simulink model "IEEE9_case"  (R2024b)
settings: Solver=FixedStepAuto  StartTime=0  StopTime=5  FixedStep=1e-7  RelTol=1e-3
values from neighbouring files (symbols this model uses):
  SG_D_1_D = 0.01056    [IEEE9_case_parameters.m]    (also in case1_parameters.m; case2_parameters.m; case3_parameters.m; case4_parameters.m)
  SG_D_1_EnableSaturation = 0    [IEEE9_case_parameters.m]    (also in case1_parameters.m; case2_parameters.m; case3_parameters.m; case4_parameters.m)
  SG_D_1_f0 = 60    [IEEE9_case_parameters.m]    (also in case1_parameters.m; case2_parameters.m; case3_parameters.m; case4_parameters.m)
  SG_D_1_H = 7.5    [IEEE9_case_parameters.m]    (also in case1_parameters.m; case2_parameters.m; case3_parameters.m; case4_parameters.m)
  SG_D_1_K_A = 20    [IEEE9_case_parameters.m]    (also in case1_parameters.m; case2_parameters.m; case3_parameters.m; case4_parameters.m)
  SG_D_1_K_E = 1.000000e+1    (= 10)    [IEEE9_case_parameters.m]    (also in case1_parameters.m; case2_parameters.m; case3_parameters.m; case4_parameters.m)
  SG_D_1_K_F = 2.363    [IEEE9_case_parameters.m]    (also in case1_parameters.m; case2_parameters.m; case3_parameters.m; case4_parameters.m)
  SG_D_1_K_s = 0.5    [IEEE9_case_parameters.m]    (also in case1_parameters.m = 5; case2_parameters.m = 5; case3_parameters.m = 5; case4_parameters.m = 5)
  SG_D_1_R_a = 0.001088    [IEEE9_case_parameters.m]    (also in case1_parameters.m; case2_parameters.m; case3_parameters.m; case4_parameters.m)
  SG_D_1_S_A = 1    [IEEE9_case_parameters.m]    (also in case1_parameters.m; case2_parameters.m; case3_parameters.m; case4_parameters.m)
  SG_D_1_S_B = 0.103    [IEEE9_case_parameters.m]    (also in case1_parameters.m; case2_parameters.m; case3_parameters.m; case4_parameters.m)
  SG_D_1_S_N = 10.659857    [IEEE9_case_parameters.m]    (also in case1_parameters.m; case2_parameters.m; case3_parameters.m; case4_parameters.m)
  SG_D_1_SpeedPara = 200    [IEEE9_case_parameters.m]    (also in case1_parameters.m; case2_parameters.m; case3_parameters.m; case4_parameters.m)
  SG_D_1_T_0 = 0.720173    [IEEE9_case_parameters.m]    (also in case1_parameters.m = 0.755522; case2_parameters.m = 0.808931; case3_parameters.m = 0.869402; case4_parameters.m = 0.729316)
  SG_D_1_T_1 = 0.3    [IEEE9_case_parameters.m]    (also in case1_parameters.m; case2_parameters.m; case3_parameters.m; case4_parameters.m)
  SG_D_1_T_2 = 0.05    [IEEE9_case_parameters.m]    (also in case1_parameters.m; case2_parameters.m; case3_parameters.m; case4_parameters.m)
  SG_D_1_T_3 = 0.02    [IEEE9_case_parameters.m]    (also in case1_parameters.m; case2_parameters.m; case3_parameters.m; case4_parameters.m)
  SG_D_1_T_4 = 0.005    [IEEE9_case_parameters.m]    (also in case1_parameters.m; case2_parameters.m; case3_parameters.m; case4_parameters.m)
  SG_D_1_T_A = 0.02    [IEEE9_case_parameters.m]    (also in case1_parameters.m; case2_parameters.m; case3_parameters.m; case4_parameters.m)
  SG_D_1_T_dd = 8.000000e+0    (= 8)    [IEEE9_case_parameters.m]    (also in case1_parameters.m; case2_parameters.m; case3_parameters.m; case4_parameters.m)
  SG_D_1_T_ddd = 0.04    [IEEE9_case_parameters.m]    (also in case1_parameters.m; case2_parameters.m; case3_parameters.m; case4_parameters.m)
  SG_D_1_T_E = 0.314    [IEEE9_case_parameters.m]    (also in case1_parameters.m; case2_parameters.m; case3_parameters.m; case4_parameters.m)
  SG_D_1_T_F = 0.35    [IEEE9_case_parameters.m]    (also in case1_parameters.m; case2_parameters.m; case3_parameters.m; case4_parameters.m)
  SG_D_1_T_qd = 0.8    [IEEE9_case_parameters.m]    (also in case1_parameters.m; case2_parameters.m; case3_parameters.m; case4_parameters.m)
  SG_D_1_T_qdd = 0.02    [IEEE9_case_parameters.m]    (also in case1_parameters.m; case2_parameters.m; case3_parameters.m; case4_parameters.m)
  SG_D_1_T_speed = 0.1    [IEEE9_case_parameters.m]    (also in case1_parameters.m = 200; case2_parameters.m = 200; case3_parameters.m = 200; case4_parameters.m = 200)
  SG_D_1_T_w = 0.5    [IEEE9_case_parameters.m]    (also in case1_parameters.m; case2_parameters.m; case3_parameters.m; case4_parameters.m)
  SG_D_1_V_ref = 1.990276    [IEEE9_case_parameters.m]    (also in case1_parameters.m = 2.042296; case2_parameters.m = 2.051388; case3_parameters.m = 2.089584; case4_parameters.m = 2.01845)
  SG_D_1_w_ref = 376.991118    [IEEE9_case_parameters.m]    (also in case1_parameters.m; case2_parameters.m; case3_parameters.m; case4_parameters.m)
  SG_D_1_wb = 6.000000e+1    (= 60)    [IEEE9_case_parameters.m]    (also in case1_parameters.m; case2_parameters.m; case3_parameters.m; case4_parameters.m)
  SG_D_1_x_d = 1.9    [IEEE9_case_parameters.m]    (also in case1_parameters.m; case2_parameters.m; case3_parameters.m; case4_parameters.m)
  SG_D_1_x_dd = 0.302    [IEEE9_case_parameters.m]    (also in case1_parameters.m; case2_parameters.m; case3_parameters.m; case4_parameters.m)
  SG_D_1_x_ddd = 0.204    [IEEE9_case_parameters.m]    (also in case1_parameters.m; case2_parameters.m; case3_parameters.m; case4_parameters.m)
  SG_D_1_x_l = 0.05    [IEEE9_case_parameters.m]    (also in case1_parameters.m; case2_parameters.m; case3_parameters.m; case4_parameters.m)
  SG_D_1_x_q = 1.3    [IEEE9_case_parameters.m]    (also in case1_parameters.m; case2_parameters.m; case3_parameters.m; case4_parameters.m)
  SG_D_1_x_qd = 0.5    [IEEE9_case_parameters.m]    (also in case1_parameters.m; case2_parameters.m; case3_parameters.m; case4_parameters.m)
  SG_D_1_x_qdd = 0.3    [IEEE9_case_parameters.m]    (also in case1_parameters.m; case2_parameters.m; case3_parameters.m; case4_parameters.m)
  SG_D_2_D = 0.02    [IEEE9_case_parameters.m]    (also in case1_parameters.m; case2_parameters.m; case3_parameters.m; case4_parameters.m)
  SG_D_2_EnableSaturation = 0    [IEEE9_case_parameters.m]    (also in case1_parameters.m; case2_parameters.m; case3_parameters.m; case4_parameters.m)
  SG_D_2_f0 = 60    [IEEE9_case_parameters.m]    (also in case1_parameters.m; case2_parameters.m; case3_parameters.m; case4_parameters.m)
  SG_D_2_H = 8.000000e+0    (= 8)    [IEEE9_case_parameters.m]    (also in case1_parameters.m; case2_parameters.m; case3_parameters.m; case4_parameters.m)
  SG_D_2_K_A = 20    [IEEE9_case_parameters.m]    (also in case1_parameters.m; case2_parameters.m; case3_parameters.m; case4_parameters.m)
  SG_D_2_K_E = 1.000000e+1    (= 10)    [IEEE9_case_parameters.m]    (also in case1_parameters.m; case2_parameters.m; case3_parameters.m; case4_parameters.m)
  SG_D_2_K_F = 2.363    [IEEE9_case_parameters.m]    (also in case1_parameters.m; case2_parameters.m; case3_parameters.m; case4_parameters.m)
  SG_D_2_K_s = 0.5    [IEEE9_case_parameters.m]    (also in case1_parameters.m = 4; case2_parameters.m = 4; case3_parameters.m = 4; case4_parameters.m = 4)
  SG_D_2_R_a = 0.001088    [IEEE9_case_parameters.m]    (also in case1_parameters.m; case2_parameters.m; case3_parameters.m; case4_parameters.m)
  SG_D_2_S_A = 1    [IEEE9_case_parameters.m]    (also in case1_parameters.m; case2_parameters.m; case3_parameters.m; case4_parameters.m)
  SG_D_2_S_B = 0.103    [IEEE9_case_parameters.m]    (also in case1_parameters.m; case2_parameters.m; case3_parameters.m; case4_parameters.m)
  SG_D_2_S_N = 10.659857    [IEEE9_case_parameters.m]    (also in case1_parameters.m; case2_parameters.m; case3_parameters.m; case4_parameters.m)
  SG_D_2_SpeedPara = 200    [IEEE9_case_parameters.m]    (also in case1_parameters.m; case2_parameters.m; case3_parameters.m; case4_parameters.m)
  SG_D_2_T_0 = 1.632913    [IEEE9_case_parameters.m]    (also in case1_parameters.m = 1.632925; case2_parameters.m = 1.632915; case3_parameters.m = 1.632914; case4_parameters.m = 1.632927)
  SG_D_2_T_1 = 0.2    [IEEE9_case_parameters.m]    (also in case1_parameters.m; case2_parameters.m; case3_parameters.m; case4_parameters.m)
  SG_D_2_T_2 = 0.05    [IEEE9_case_parameters.m]    (also in case1_parameters.m; case2_parameters.m; case3_parameters.m; case4_parameters.m)
  SG_D_2_T_3 = 0.02    [IEEE9_case_parameters.m]    (also in case1_parameters.m; case2_parameters.m; case3_parameters.m; case4_parameters.m)
  SG_D_2_T_4 = 0.005    [IEEE9_case_parameters.m]    (also in case1_parameters.m; case2_parameters.m; case3_parameters.m; case4_parameters.m)
  SG_D_2_T_A = 0.02    [IEEE9_case_parameters.m]    (also in case1_parameters.m; case2_parameters.m; case3_parameters.m; case4_parameters.m)
  SG_D_2_T_dd = 7.9    [IEEE9_case_parameters.m]    (also in case1_parameters.m; case2_parameters.m; case3_parameters.m; case4_parameters.m)
  SG_D_2_T_ddd = 0.04    [IEEE9_case_parameters.m]    (also in case1_parameters.m; case2_parameters.m; case3_parameters.m; case4_parameters.m)
  SG_D_2_T_E = 0.314    [IEEE9_case_parameters.m]    (also in case1_parameters.m; case2_parameters.m; case3_parameters.m; case4_parameters.m)
  SG_D_2_T_F = 0.35    [IEEE9_case_parameters.m]    (also in case1_parameters.m; case2_parameters.m; case3_parameters.m; case4_parameters.m)
  SG_D_2_T_qd = 0.8    [IEEE9_case_parameters.m]    (also in case1_parameters.m; case2_parameters.m; case3_parameters.m; case4_parameters.m)
  SG_D_2_T_qdd = 0.015    [IEEE9_case_parameters.m]    (also in case1_parameters.m; case2_parameters.m; case3_parameters.m; case4_parameters.m)
  SG_D_2_T_speed = 0.1    [IEEE9_case_parameters.m]    (also in case1_parameters.m = 150; case2_parameters.m = 150; case3_parameters.m = 150; case4_parameters.m = 150)
  SG_D_2_T_w = 0.35    [IEEE9_case_parameters.m]    (also in case1_parameters.m; case2_parameters.m; case3_parameters.m; case4_parameters.m)
  SG_D_2_V_ref = 2.58547    [IEEE9_case_parameters.m]    (also in case1_parameters.m = 2.597896; case2_parameters.m = 2.587136; case3_parameters.m = 2.586042; case4_parameters.m = 2.599679)
  SG_D_2_w_ref = 376.991118    [IEEE9_case_parameters.m]    (also in case1_parameters.m; case2_parameters.m; case3_parameters.m; case4_parameters.m)
  SG_D_2_wb = 6.000000e+1    (= 60)    [IEEE9_case_parameters.m]    (also in case1_parameters.m; case2_parameters.m; case3_parameters.m; case4_parameters.m)
  SG_D_2_x_d = 1.8    [IEEE9_case_parameters.m]    (also in case1_parameters.m; case2_parameters.m; case3_parameters.m; case4_parameters.m)
  SG_D_2_x_dd = 0.302    [IEEE9_case_parameters.m]    (also in case1_parameters.m; case2_parameters.m; case3_parameters.m; case4_parameters.m)
  SG_D_2_x_ddd = 0.204    [IEEE9_case_parameters.m]    (also in case1_parameters.m; case2_parameters.m; case3_parameters.m; case4_parameters.m)
  SG_D_2_x_l = 0.05    [IEEE9_case_parameters.m]    (also in case1_parameters.m; case2_parameters.m; case3_parameters.m; case4_parameters.m)
  SG_D_2_x_q = 1.25    [IEEE9_case_parameters.m]    (also in case1_parameters.m; case2_parameters.m; case3_parameters.m; case4_parameters.m)
  SG_D_2_x_qd = 0.5    [IEEE9_case_parameters.m]    (also in case1_parameters.m; case2_parameters.m; case3_parameters.m; case4_parameters.m)
  SG_D_2_x_qdd = 0.3    [IEEE9_case_parameters.m]    (also in case1_parameters.m; case2_parameters.m; case3_parameters.m; case4_parameters.m)
  SG_D_3_D = 0.02    [IEEE9_case_parameters.m]    (also in case1_parameters.m; case2_parameters.m; case3_parameters.m; case4_parameters.m)
  SG_D_3_EnableSaturation = 0    [IEEE9_case_parameters.m]    (also in case1_parameters.m; case2_parameters.m; case3_parameters.m; case4_parameters.m)
  SG_D_3_f0 = 60    [IEEE9_case_parameters.m]    (also in case1_parameters.m; case2_parameters.m; case3_parameters.m; case4_parameters.m)
  SG_D_3_H = 7.7    [IEEE9_case_parameters.m]    (also in case1_parameters.m; case2_parameters.m; case3_parameters.m; case4_parameters.m)
  SG_D_3_K_A = 20    [IEEE9_case_parameters.m]    (also in case1_parameters.m; case2_parameters.m; case3_parameters.m; case4_parameters.m)
  SG_D_3_K_E = 1.000000e+1    (= 10)    [IEEE9_case_parameters.m]    (also in case1_parameters.m; case2_parameters.m; case3_parameters.m; case4_parameters.m)
  SG_D_3_K_F = 2.363    [IEEE9_case_parameters.m]    (also in case1_parameters.m; case2_parameters.m; case3_parameters.m; case4_parameters.m)
  SG_D_3_K_s = 0.2    [IEEE9_case_parameters.m]    (also in case1_parameters.m = 2; case2_parameters.m = 2; case3_parameters.m = 2; case4_parameters.m = 2)
  SG_D_3_R_a = 0.001088    [IEEE9_case_parameters.m]    (also in case1_parameters.m; case2_parameters.m; case3_parameters.m; case4_parameters.m)
  SG_D_3_S_A = 1    [IEEE9_case_parameters.m]    (also in case1_parameters.m; case2_parameters.m; case3_parameters.m; case4_parameters.m)
  SG_D_3_S_B = 0.103    [IEEE9_case_parameters.m]    (also in case1_parameters.m; case2_parameters.m; case3_parameters.m; case4_parameters.m)
  SG_D_3_S_N = 10.659857    [IEEE9_case_parameters.m]    (also in case1_parameters.m; case2_parameters.m; case3_parameters.m; case4_parameters.m)
  SG_D_3_SpeedPara = 200    [IEEE9_case_parameters.m]    (also in case1_parameters.m; case2_parameters.m; case3_parameters.m; case4_parameters.m)
  SG_D_3_T_0 = 0.850788    [IEEE9_case_parameters.m]    (also in case1_parameters.m = 0.850786; case2_parameters.m = 0.850787; case3_parameters.m; case4_parameters.m = 0.850786)
  SG_D_3_T_1 = 0.2    [IEEE9_case_parameters.m]    (also in case1_parameters.m; case2_parameters.m; case3_parameters.m; case4_parameters.m)
  SG_D_3_T_2 = 0.05    [IEEE9_case_parameters.m]    (also in case1_parameters.m; case2_parameters.m; case3_parameters.m; case4_parameters.m)
  SG_D_3_T_3 = 0.02    [IEEE9_case_parameters.m]    (also in case1_parameters.m; case2_parameters.m; case3_parameters.m; case4_parameters.m)
  SG_D_3_T_4 = 0.005    [IEEE9_case_parameters.m]    (also in case1_parameters.m; case2_parameters.m; case3_parameters.m; case4_parameters.m)
  SG_D_3_T_A = 0.02    [IEEE9_case_parameters.m]    (also in case1_parameters.m; case2_parameters.m; case3_parameters.m; case4_parameters.m)
  SG_D_3_T_dd = 8.1    [IEEE9_case_parameters.m]    (also in case1_parameters.m; case2_parameters.m; case3_parameters.m; case4_parameters.m)
  SG_D_3_T_ddd = 0.04    [IEEE9_case_parameters.m]    (also in case1_parameters.m; case2_parameters.m; case3_parameters.m; case4_parameters.m)
  SG_D_3_T_E = 0.314    [IEEE9_case_parameters.m]    (also in case1_parameters.m; case2_parameters.m; case3_parameters.m; case4_parameters.m)
  SG_D_3_T_F = 0.35    [IEEE9_case_parameters.m]    (also in case1_parameters.m; case2_parameters.m; case3_parameters.m; case4_parameters.m)
  SG_D_3_T_qd = 0.8    [IEEE9_case_parameters.m]    (also in case1_parameters.m; case2_parameters.m; case3_parameters.m; case4_parameters.m)
  SG_D_3_T_qdd = 0.015    [IEEE9_case_parameters.m]    (also in case1_parameters.m; case2_parameters.m; case3_parameters.m; case4_parameters.m)
  SG_D_3_T_speed = 0.1    [IEEE9_case_parameters.m]    (also in case1_parameters.m = 180; case2_parameters.m = 180; case3_parameters.m = 180; case4_parameters.m = 180)
  SG_D_3_T_w = 0.4    [IEEE9_case_parameters.m]    (also in case1_parameters.m; case2_parameters.m; case3_parameters.m; case4_parameters.m)
  SG_D_3_V_ref = 1.892727    [IEEE9_case_parameters.m]    (also in case1_parameters.m = 1.906439; case2_parameters.m = 1.895535; case3_parameters.m = 1.892105; case4_parameters.m = 1.906598)
  SG_D_3_w_ref = 376.991118    [IEEE9_case_parameters.m]    (also in case1_parameters.m; case2_parameters.m; case3_parameters.m; case4_parameters.m)
  SG_D_3_wb = 6.000000e+1    (= 60)    [IEEE9_case_parameters.m]    (also in case1_parameters.m; case2_parameters.m; case3_parameters.m; case4_parameters.m)
  SG_D_3_x_d = 1.85    [IEEE9_case_parameters.m]    (also in case1_parameters.m; case2_parameters.m; case3_parameters.m; case4_parameters.m)
  SG_D_3_x_dd = 0.302    [IEEE9_case_parameters.m]    (also in case1_parameters.m; case2_parameters.m; case3_parameters.m; case4_parameters.m)
  SG_D_3_x_ddd = 0.204    [IEEE9_case_parameters.m]    (also in case1_parameters.m; case2_parameters.m; case3_parameters.m; case4_parameters.m)
  SG_D_3_x_l = 0.05    [IEEE9_case_parameters.m]    (also in case1_parameters.m; case2_parameters.m; case3_parameters.m; case4_parameters.m)
  SG_D_3_x_q = 1.2    [IEEE9_case_parameters.m]    (also in case1_parameters.m; case2_parameters.m; case3_parameters.m; case4_parameters.m)
  SG_D_3_x_qd = 0.5    [IEEE9_case_parameters.m]    (also in case1_parameters.m; case2_parameters.m; case3_parameters.m; case4_parameters.m)
  SG_D_3_x_qdd = 0.3    [IEEE9_case_parameters.m]    (also in case1_parameters.m; case2_parameters.m; case3_parameters.m; case4_parameters.m)
(part 2 of 12)

== system IEEE9_case/SG_D_2 ==
  v_d_SG_D_2 : Inport
  v_q_SG_D_2 : Inport  Port=2
  E_fd_SG_D_2 : Integrator  InitialCondition=3.1709404313191003
  Px_1_SG_D_2 : Integrator  InitialCondition=0.0
  Px_2_SG_D_2 : Integrator  InitialCondition=0.0
  Px_3_SG_D_2 : Integrator  InitialCondition=1.4014353908316667e-25
  R_f_SG_D_2 : Integrator  InitialCondition=21.408377826305813
  T_e_SG_D_2_block : Subsystem
  T_m_SG_D_2 : Integrator  InitialCondition=1.6329134567527237
  V_f_SG_D_2 : Integrator  InitialCondition=31.709404313191
  d_E_fd_SG_D_2_block : Subsystem
  d_Px_1_SG_D_2_block : Subsystem
  d_Px_2_SG_D_2_block : Subsystem
  d_Px_3_SG_D_2_block : Subsystem
  d_R_f_SG_D_2_block : Subsystem
  d_T_m_SG_D_2_block : Subsystem
  d_V_f_SG_D_2_block : Subsystem
  d_psi_1d_SG_D_2_block : Subsystem
  d_psi_d_SG_D_2_block : Subsystem
  d_psi_fd_SG_D_2_block : Subsystem
  d_psi_gq_SG_D_2_block : Subsystem
  d_psi_kq_SG_D_2_block : Subsystem
  d_psi_q_SG_D_2_block : Subsystem
  d_theta_SG_D_2_block : Subsystem
  d_w_SG_D_2_block : Subsystem
  i_d_SG_D_2_block : Subsystem
  i_q_SG_D_2_block : Subsystem
  psi_1d_SG_D_2 : Integrator  InitialCondition=0.5768638700038088
  psi_d_SG_D_2 : Integrator  InitialCondition=0.5027473968233718
  psi_fd_SG_D_2 : Integrator  InitialCondition=0.9504108948332107
  psi_gq_SG_D_2 : Integrator  InitialCondition=0.519890601695655
  psi_kq_SG_D_2 : Integrator  InitialCondition=-0.8318249627130481
  psi_q_SG_D_2 : Integrator  InitialCondition=-0.8664843361594251
  theta_SG_D_2 : Integrator  InitialCondition=1.2136458258562681
  theta_SG_D_2_out_block : Subsystem
  w_SG_D_2 : Integrator  InitialCondition=376.99111843077515
  w_SG_D_2_out_block : Subsystem
  i_d_SG_D_2 : Outport
  i_q_SG_D_2 : Outport  Port=2
  T_e_SG_D_2 : Outport  Port=3
  w_SG_D_2_out : Outport  Port=4
  theta_SG_D_2_out : Outport  Port=5
  wires:
  T_e_SG_D_2_block/1(Blockout_T_e_SG_D_2_66ce8) -> T_e_SG_D_2/1
  d_Px_2_SG_D_2_block/1(Blockout_d_Px_2_SG_D_2_a6ada) -> Px_2_SG_D_2/1
  d_T_m_SG_D_2_block/1(Blockout_d_T_m_SG_D_2_0f7e5) -> T_m_SG_D_2/1
  w_SG_D_2/1 -> d_psi_q_SG_D_2_block/9(State_w_SG_D_2_e3f21), d_psi_d_SG_D_2_block/9(State_w_SG_D_2_4590a), d_w_SG_D_2_block/1(State_w_SG_D_2_d930b), d_V_f_SG_D_2_block/8(State_w_SG_D_2_abcad), d_V_f_SG_D_2_block/13(State_w_SG_D_2_ea831), d_T_m_SG_D_2_block/1(State_w_SG_D_2_27a0d), d_Px_2_SG_D_2_block/4(State_w_SG_D_2_c021f), d_Px_3_SG_D_2_block/6(State_w_SG_D_2_71684), d_theta_SG_D_2_block/1(State_w_SG_D_2_1f89c), w_SG_D_2_out_block/1(State_w_SG_D_2_bfe63), d_Px_1_SG_D_2_block/2(State_w_SG_D_2_d8062)
  d_Px_1_SG_D_2_block/1(Blockout_d_Px_1_SG_D_2_5e8fa) -> Px_1_SG_D_2/1
  psi_fd_SG_D_2/1 -> d_psi_fd_SG_D_2_block/2(State_psi_fd_SG_D_2_96da5), d_psi_fd_SG_D_2_block/4(State_psi_fd_SG_D_2_18c77), d_psi_fd_SG_D_2_block/10(State_psi_fd_SG_D_2_7bfa6), d_psi_d_SG_D_2_block/3(State_psi_fd_SG_D_2_6b3f8), d_w_SG_D_2_block/10(State_psi_fd_SG_D_2_8df94), d_psi_1d_SG_D_2_block/5(State_psi_fd_SG_D_2_1a1ec), d_V_f_SG_D_2_block/6(State_psi_fd_SG_D_2_e00a4), d_psi_fd_SG_D_2_block/7(State_psi_fd_SG_D_2_4a3c7), i_d_SG_D_2_block/7(State_psi_fd_SG_D_2_83be3), i_q_SG_D_2_block/7(State_psi_fd_SG_D_2_97667), d_psi_1d_SG_D_2_block/2(State_psi_fd_SG_D_2_683d9), T_e_SG_D_2_block/8(State_psi_fd_SG_D_2_499b8)
  d_Px_3_SG_D_2_block/1(Blockout_d_Px_3_SG_D_2_2df83) -> Px_3_SG_D_2/1
  psi_q_SG_D_2/1 -> d_psi_q_SG_D_2_block/3(State_psi_q_SG_D_2_c5dff), d_psi_gq_SG_D_2_block/6(State_psi_q_SG_D_2_75609), d_psi_gq_SG_D_2_block/9(State_psi_q_SG_D_2_7ca39), d_psi_kq_SG_D_2_block/5(State_psi_q_SG_D_2_cf35f), d_w_SG_D_2_block/7(State_psi_q_SG_D_2_7c783), i_d_SG_D_2_block/3(State_psi_q_SG_D_2_90cca), d_V_f_SG_D_2_block/11(State_psi_q_SG_D_2_5bd97), d_w_SG_D_2_block/6(State_psi_q_SG_D_2_33516), i_q_SG_D_2_block/3(State_psi_q_SG_D_2_067b4), T_e_SG_D_2_block/4(State_psi_q_SG_D_2_b203e), d_V_f_SG_D_2_block/7(State_psi_q_SG_D_2_52f21), d_psi_d_SG_D_2_block/8(State_psi_q_SG_D_2_03603), T_e_SG_D_2_block/5(State_psi_q_SG_D_2_f483f)
  w_SG_D_2_out_block/1(Blockout_w_SG_D_2_out_ddf0a) -> w_SG_D_2_out/1
  d_theta_SG_D_2_block/1(Blockout_d_theta_SG_D_2_e52e5) -> theta_SG_D_2/1
  Px_1_SG_D_2/1 -> d_Px_1_SG_D_2_block/1(State_Px_1_SG_D_2_4c7b1), d_Px_2_SG_D_2_block/2(State_Px_1_SG_D_2_be7f9), d_Px_2_SG_D_2_block/3(State_Px_1_SG_D_2_fde36), d_Px_3_SG_D_2_block/5(State_Px_1_SG_D_2_44be4), d_Px_3_SG_D_2_block/4(State_Px_1_SG_D_2_79294)
  psi_kq_SG_D_2/1 -> d_psi_q_SG_D_2_block/2(State_psi_kq_SG_D_2_3ead0), d_psi_gq_SG_D_2_block/5(State_psi_kq_SG_D_2_ca188), d_psi_gq_SG_D_2_block/8(State_psi_kq_SG_D_2_03d84), d_psi_kq_SG_D_2_block/4(State_psi_kq_SG_D_2_d1d79), d_psi_kq_SG_D_2_block/2(State_psi_kq_SG_D_2_6c00b), d_psi_gq_SG_D_2_block/3(State_psi_kq_SG_D_2_80cf3), d_V_f_SG_D_2_block/10(State_psi_kq_SG_D_2_f7c2b), i_d_SG_D_2_block/2(State_psi_kq_SG_D_2_22efa), i_q_SG_D_2_block/2(State_psi_kq_SG_D_2_62e42), d_w_SG_D_2_block/5(State_psi_kq_SG_D_2_3606b), T_e_SG_D_2_block/3(State_psi_kq_SG_D_2_3e69f)
  theta_SG_D_2/1 -> d_psi_d_SG_D_2_block/5(State_theta_SG_D_2_d1f6e), d_psi_q_SG_D_2_block/7(State_theta_SG_D_2_bef8f), i_d_SG_D_2_block/8(State_theta_SG_D_2_1b926), i_d_SG_D_2_block/4(State_theta_SG_D_2_b69be), i_q_SG_D_2_block/8(State_theta_SG_D_2_5175d), i_q_SG_D_2_block/4(State_theta_SG_D_2_eabbf), d_psi_d_SG_D_2_block/7(State_theta_SG_D_2_8a255), theta_SG_D_2_out_block/1(State_theta_SG_D_2_b5c4c), d_psi_q_SG_D_2_block/5(State_theta_SG_D_2_4da9a)
  v_d_SG_D_2/1 -> d_psi_d_SG_D_2_block/4(Input_v_d_SG_D_2_43371), d_psi_q_SG_D_2_block/4(Input_v_d_SG_D_2_9bfd5)
  d_V_f_SG_D_2_block/1(Blockout_d_V_f_SG_D_2_b7af1) -> V_f_SG_D_2/1
  v_q_SG_D_2/1 -> d_psi_d_SG_D_2_block/6(Input_v_q_SG_D_2_68fd3), d_psi_q_SG_D_2_block/6(Input_v_q_SG_D_2_22342)
  T_m_SG_D_2/1 -> d_T_m_SG_D_2_block/2(State_T_m_SG_D_2_c6b35), d_w_SG_D_2_block/2(State_T_m_SG_D_2_4121b)
  Px_2_SG_D_2/1 -> d_Px_2_SG_D_2_block/1(State_Px_2_SG_D_2_06eab), d_Px_3_SG_D_2_block/2(State_Px_2_SG_D_2_44f04), d_Px_3_SG_D_2_block/3(State_Px_2_SG_D_2_acc18)
  psi_1d_SG_D_2/1 -> d_psi_fd_SG_D_2_block/3(State_psi_1d_SG_D_2_c35a5), d_psi_fd_SG_D_2_block/5(State_psi_1d_SG_D_2_e2991), d_psi_fd_SG_D_2_block/8(State_psi_1d_SG_D_2_7e692), d_psi_d_SG_D_2_block/1(State_psi_1d_SG_D_2_9e75a), d_psi_1d_SG_D_2_block/1(State_psi_1d_SG_D_2_41588), d_psi_1d_SG_D_2_block/3(State_psi_1d_SG_D_2_bbec1), d_w_SG_D_2_block/8(State_psi_1d_SG_D_2_76690), i_d_SG_D_2_block/5(State_psi_1d_SG_D_2_5d51d), T_e_SG_D_2_block/6(State_psi_1d_SG_D_2_95086), i_q_SG_D_2_block/5(State_psi_1d_SG_D_2_50cf4), d_V_f_SG_D_2_block/4(State_psi_1d_SG_D_2_a6b10)
  psi_gq_SG_D_2/1 -> d_psi_q_SG_D_2_block/1(State_psi_gq_SG_D_2_c07ab), d_psi_gq_SG_D_2_block/1(State_psi_gq_SG_D_2_f5a80), d_psi_gq_SG_D_2_block/2(State_psi_gq_SG_D_2_b3a61), d_psi_gq_SG_D_2_block/4(State_psi_gq_SG_D_2_c36e1), d_psi_kq_SG_D_2_block/3(State_psi_gq_SG_D_2_ad537), d_w_SG_D_2_block/4(State_psi_gq_SG_D_2_b8927), d_psi_kq_SG_D_2_block/1(State_psi_gq_SG_D_2_d035b), d_V_f_SG_D_2_block/9(State_psi_gq_SG_D_2_8793d), i_d_SG_D_2_block/1(State_psi_gq_SG_D_2_c758c), i_q_SG_D_2_block/1(State_psi_gq_SG_D_2_0dc4e), T_e_SG_D_2_block/2(State_psi_gq_SG_D_2_748c1), d_psi_gq_SG_D_2_block/7(State_psi_gq_SG_D_2_ee37c)
  i_d_SG_D_2_block/1(Blockout_i_d_SG_D_2_05ed7) -> i_d_SG_D_2/1
  psi_d_SG_D_2/1 -> d_psi_fd_SG_D_2_block/6(State_psi_d_SG_D_2_08540), d_psi_fd_SG_D_2_block/9(State_psi_d_SG_D_2_798aa), d_psi_d_SG_D_2_block/2(State_psi_d_SG_D_2_1509d), d_psi_q_SG_D_2_block/8(State_psi_d_SG_D_2_94ada), d_psi_1d_SG_D_2_block/4(State_psi_d_SG_D_2_88e69), d_w_SG_D_2_block/9(State_psi_d_SG_D_2_d8055), d_V_f_SG_D_2_block/12(State_psi_d_SG_D_2_b502c), i_d_SG_D_2_block/6(State_psi_d_SG_D_2_f7721), d_V_f_SG_D_2_block/5(State_psi_d_SG_D_2_4cd87), d_w_SG_D_2_block/3(State_psi_d_SG_D_2_dbd57), i_q_SG_D_2_block/6(State_psi_d_SG_D_2_5901a), T_e_SG_D_2_block/1(State_psi_d_SG_D_2_ab5a2), T_e_SG_D_2_block/7(State_psi_d_SG_D_2_9e58e)
  d_R_f_SG_D_2_block/1(Blockout_d_R_f_SG_D_2_96516) -> R_f_SG_D_2/1
  R_f_SG_D_2/1 -> d_V_f_SG_D_2_block/2(State_R_f_SG_D_2_2cf24), d_R_f_SG_D_2_block/2(State_R_f_SG_D_2_17e2e)
  theta_SG_D_2_out_block/1(Blockout_theta_SG_D_2_out_8a415) -> theta_SG_D_2_out/1
  d_psi_kq_SG_D_2_block/1(Blockout_d_psi_kq_SG_D_2_39ae4) -> psi_kq_SG_D_2/1
  i_q_SG_D_2_block/1(Blockout_i_q_SG_D_2_9bb23) -> i_q_SG_D_2/1
  d_psi_q_SG_D_2_block/1(Blockout_d_psi_q_SG_D_2_d035a) -> psi_q_SG_D_2/1
  d_psi_d_SG_D_2_block/1(Blockout_d_psi_d_SG_D_2_65f41) -> psi_d_SG_D_2/1
  d_w_SG_D_2_block/1(Blockout_d_w_SG_D_2_07836) -> w_SG_D_2/1
  d_psi_gq_SG_D_2_block/1(Blockout_d_psi_gq_SG_D_2_ad782) -> psi_gq_SG_D_2/1
  d_psi_1d_SG_D_2_block/1(Blockout_d_psi_1d_SG_D_2_e4c33) -> psi_1d_SG_D_2/1
  Px_3_SG_D_2/1 -> d_V_f_SG_D_2_block/3(State_Px_3_SG_D_2_f8af3), d_Px_3_SG_D_2_block/1(State_Px_3_SG_D_2_e98da)
  V_f_SG_D_2/1 -> d_V_f_SG_D_2_block/14(State_V_f_SG_D_2_c3639), d_E_fd_SG_D_2_block/2(State_V_f_SG_D_2_a732e)
  d_E_fd_SG_D_2_block/1(Blockout_d_E_fd_SG_D_2_9aa5a) -> E_fd_SG_D_2/1
  E_fd_SG_D_2/1 -> d_R_f_SG_D_2_block/1(State_E_fd_SG_D_2_c2b5e), d_E_fd_SG_D_2_block/1(State_E_fd_SG_D_2_1a251), d_psi_fd_SG_D_2_block/1(State_E_fd_SG_D_2_7c2d9), d_V_f_SG_D_2_block/1(State_E_fd_SG_D_2_94712)
  d_psi_fd_SG_D_2_block/1(Blockout_d_psi_fd_SG_D_2_fb63c) -> psi_fd_SG_D_2/1

== system IEEE9_case/SG_D_3 ==
  v_d_SG_D_3 : Inport
  v_q_SG_D_3 : Inport  Port=2
  E_fd_SG_D_3 : Integrator  InitialCondition=1.7854541179534191
  Px_1_SG_D_3 : Integrator  InitialCondition=0.0
  Px_2_SG_D_3 : Integrator  InitialCondition=0.0
  Px_3_SG_D_3 : Integrator  InitialCondition=-3.646179370485784e-25
  R_f_SG_D_3 : Integrator  InitialCondition=12.054365944925513
  T_e_SG_D_3_block : Subsystem
  T_m_SG_D_3 : Integrator  InitialCondition=0.8507875290299154
  V_f_SG_D_3 : Integrator  InitialCondition=17.85454117953419
  d_E_fd_SG_D_3_block : Subsystem
  d_Px_1_SG_D_3_block : Subsystem
  d_Px_2_SG_D_3_block : Subsystem
  d_Px_3_SG_D_3_block : Subsystem
  d_R_f_SG_D_3_block : Subsystem
  d_T_m_SG_D_3_block : Subsystem
  d_V_f_SG_D_3_block : Subsystem
  d_psi_1d_SG_D_3_block : Subsystem
  d_psi_d_SG_D_3_block : Subsystem
  d_psi_fd_SG_D_3_block : Subsystem
  d_psi_gq_SG_D_3_block : Subsystem
  d_psi_kq_SG_D_3_block : Subsystem
  d_psi_q_SG_D_3_block : Subsystem
  d_theta_SG_D_3_block : Subsystem
  d_w_SG_D_3_block : Subsystem
  i_d_SG_D_3_block : Subsystem
  i_q_SG_D_3_block : Subsystem
  psi_1d_SG_D_3 : Integrator  InitialCondition=0.7146699663821662
  psi_d_SG_D_3 : Integrator  InitialCondition=0.6849259621718535
  psi_fd_SG_D_3 : Integrator  InitialCondition=0.8645797476021416
  psi_gq_SG_D_3 : Integrator  InitialCondition=0.4257641600475868
  psi_kq_SG_D_3 : Integrator  InitialCondition=-0.6994696915067499
  psi_q_SG_D_3 : Integrator  InitialCondition=-0.7298814172244347
  theta_SG_D_3 : Integrator  InitialCondition=0.9004730426917992
  theta_SG_D_3_out_block : Subsystem
  w_SG_D_3 : Integrator  InitialCondition=376.99111843077515
  w_SG_D_3_out_block : Subsystem
  i_d_SG_D_3 : Outport
  i_q_SG_D_3 : Outport  Port=2
  T_e_SG_D_3 : Outport  Port=3
  w_SG_D_3_out : Outport  Port=4
  theta_SG_D_3_out : Outport  Port=5
  wires:
  d_Px_1_SG_D_3_block/1(Blockout_d_Px_1_SG_D_3_7cdee) -> Px_1_SG_D_3/1
  w_SG_D_3/1 -> d_psi_d_SG_D_3_block/9(State_w_SG_D_3_c8b72), d_psi_q_SG_D_3_block/9(State_w_SG_D_3_7541e), d_V_f_SG_D_3_block/8(State_w_SG_D_3_2cca7), d_V_f_SG_D_3_block/13(State_w_SG_D_3_790e2), d_T_m_SG_D_3_block/1(State_w_SG_D_3_50cf4), d_w_SG_D_3_block/1(State_w_SG_D_3_22a21), d_theta_SG_D_3_block/1(State_w_SG_D_3_1039d), d_Px_1_SG_D_3_block/2(State_w_SG_D_3_88dc5), d_Px_3_SG_D_3_block/6(State_w_SG_D_3_532bc), d_Px_2_SG_D_3_block/4(State_w_SG_D_3_fe91f), w_SG_D_3_out_block/1(State_w_SG_D_3_e2767)
  R_f_SG_D_3/1 -> d_V_f_SG_D_3_block/2(State_R_f_SG_D_3_5baad), d_R_f_SG_D_3_block/2(State_R_f_SG_D_3_c9e06)
  w_SG_D_3_out_block/1(Blockout_w_SG_D_3_out_e7af9) -> w_SG_D_3_out/1
  d_Px_2_SG_D_3_block/1(Blockout_d_Px_2_SG_D_3_e1b1c) -> Px_2_SG_D_3/1
  d_w_SG_D_3_block/1(Blockout_d_w_SG_D_3_c2bca) -> w_SG_D_3/1
  Px_1_SG_D_3/1 -> d_Px_2_SG_D_3_block/2(State_Px_1_SG_D_3_30b70), d_Px_1_SG_D_3_block/1(State_Px_1_SG_D_3_67f42), d_Px_2_SG_D_3_block/3(State_Px_1_SG_D_3_0e345), d_Px_3_SG_D_3_block/5(State_Px_1_SG_D_3_f96ae), d_Px_3_SG_D_3_block/4(State_Px_1_SG_D_3_a37cd)
  d_theta_SG_D_3_block/1(Blockout_d_theta_SG_D_3_5365d) -> theta_SG_D_3/1
  psi_fd_SG_D_3/1 -> d_psi_fd_SG_D_3_block/2(State_psi_fd_SG_D_3_dfb80), d_psi_fd_SG_D_3_block/4(State_psi_fd_SG_D_3_019c6), d_psi_fd_SG_D_3_block/7(State_psi_fd_SG_D_3_c7d54), d_psi_d_SG_D_3_block/3(State_psi_fd_SG_D_3_f7fa4), d_psi_1d_SG_D_3_block/5(State_psi_fd_SG_D_3_9f125), d_psi_1d_SG_D_3_block/2(State_psi_fd_SG_D_3_cacc3), i_d_SG_D_3_block/7(State_psi_fd_SG_D_3_e8270), d_w_SG_D_3_block/10(State_psi_fd_SG_D_3_07cc6), d_psi_fd_SG_D_3_block/10(State_psi_fd_SG_D_3_c8342), i_q_SG_D_3_block/7(State_psi_fd_SG_D_3_037e3), d_V_f_SG_D_3_block/6(State_psi_fd_SG_D_3_86d68), T_e_SG_D_3_block/8(State_psi_fd_SG_D_3_e857c)
  d_Px_3_SG_D_3_block/1(Blockout_d_Px_3_SG_D_3_549f5) -> Px_3_SG_D_3/1
  d_T_m_SG_D_3_block/1(Blockout_d_T_m_SG_D_3_5f1a1) -> T_m_SG_D_3/1
  psi_gq_SG_D_3/1 -> d_psi_q_SG_D_3_block/1(State_psi_gq_SG_D_3_cf09c), d_psi_gq_SG_D_3_block/1(State_psi_gq_SG_D_3_41ff6), d_psi_gq_SG_D_3_block/4(State_psi_gq_SG_D_3_a8b01), d_psi_gq_SG_D_3_block/7(State_psi_gq_SG_D_3_e2885), d_psi_gq_SG_D_3_block/2(State_psi_gq_SG_D_3_3e973), d_psi_kq_SG_D_3_block/1(State_psi_gq_SG_D_3_86c60), d_psi_kq_SG_D_3_block/3(State_psi_gq_SG_D_3_7b374), d_w_SG_D_3_block/4(State_psi_gq_SG_D_3_862a3), d_V_f_SG_D_3_block/9(State_psi_gq_SG_D_3_817f4), i_q_SG_D_3_block/1(State_psi_gq_SG_D_3_a510d), T_e_SG_D_3_block/2(State_psi_gq_SG_D_3_6ebde), i_d_SG_D_3_block/1(State_psi_gq_SG_D_3_77a5e)
  Px_2_SG_D_3/1 -> d_Px_2_SG_D_3_block/1(State_Px_2_SG_D_3_ac8d1), d_Px_3_SG_D_3_block/3(State_Px_2_SG_D_3_7d1eb), d_Px_3_SG_D_3_block/2(State_Px_2_SG_D_3_c6c25)
  psi_kq_SG_D_3/1 -> d_psi_q_SG_D_3_block/2(State_psi_kq_SG_D_3_c8fad), d_psi_gq_SG_D_3_block/3(State_psi_kq_SG_D_3_68a0b), d_psi_gq_SG_D_3_block/5(State_psi_kq_SG_D_3_062fd), d_psi_gq_SG_D_3_block/8(State_psi_kq_SG_D_3_7f586), d_w_SG_D_3_block/5(State_psi_kq_SG_D_3_8659d), d_psi_kq_SG_D_3_block/4(State_psi_kq_SG_D_3_310cd), d_V_f_SG_D_3_block/10(State_psi_kq_SG_D_3_c6b94), i_d_SG_D_3_block/2(State_psi_kq_SG_D_3_e468d), d_psi_kq_SG_D_3_block/2(State_psi_kq_SG_D_3_0238a), i_q_SG_D_3_block/2(State_psi_kq_SG_D_3_41d81), T_e_SG_D_3_block/3(State_psi_kq_SG_D_3_8ca03)
  d_psi_kq_SG_D_3_block/1(Blockout_d_psi_kq_SG_D_3_0e0d5) -> psi_kq_SG_D_3/1
  psi_1d_SG_D_3/1 -> d_psi_fd_SG_D_3_block/3(State_psi_1d_SG_D_3_bd0db), d_psi_fd_SG_D_3_block/5(State_psi_1d_SG_D_3_eed35), d_psi_fd_SG_D_3_block/8(State_psi_1d_SG_D_3_a1855), d_psi_d_SG_D_3_block/1(State_psi_1d_SG_D_3_ec6d7), d_psi_1d_SG_D_3_block/1(State_psi_1d_SG_D_3_dcaf3), d_psi_1d_SG_D_3_block/3(State_psi_1d_SG_D_3_98130), d_w_SG_D_3_block/8(State_psi_1d_SG_D_3_9d901), d_V_f_SG_D_3_block/4(State_psi_1d_SG_D_3_130c5), i_q_SG_D_3_block/5(State_psi_1d_SG_D_3_fb8fd), T_e_SG_D_3_block/6(State_psi_1d_SG_D_3_57116), i_d_SG_D_3_block/5(State_psi_1d_SG_D_3_213a5)
  theta_SG_D_3/1 -> d_psi_d_SG_D_3_block/5(State_theta_SG_D_3_79acd), d_psi_q_SG_D_3_block/5(State_theta_SG_D_3_c9886), d_psi_q_SG_D_3_block/7(State_theta_SG_D_3_067ed), i_d_SG_D_3_block/8(State_theta_SG_D_3_fbfef), i_q_SG_D_3_block/8(State_theta_SG_D_3_9d612), i_d_SG_D_3_block/4(State_theta_SG_D_3_b7be5), d_psi_d_SG_D_3_block/7(State_theta_SG_D_3_d0ec2), theta_SG_D_3_out_block/1(State_theta_SG_D_3_72496), i_q_SG_D_3_block/4(State_theta_SG_D_3_6f7b7)
  psi_d_SG_D_3/1 -> d_psi_fd_SG_D_3_block/9(State_psi_d_SG_D_3_9ca4c), d_psi_d_SG_D_3_block/2(State_psi_d_SG_D_3_cd386), d_psi_q_SG_D_3_block/8(State_psi_d_SG_D_3_bc54d), d_psi_1d_SG_D_3_block/4(State_psi_d_SG_D_3_fbd14), d_psi_fd_SG_D_3_block/6(State_psi_d_SG_D_3_bb63b), d_w_SG_D_3_block/9(State_psi_d_SG_D_3_acc7c), d_V_f_SG_D_3_block/12(State_psi_d_SG_D_3_a8f70), i_d_SG_D_3_block/6(State_psi_d_SG_D_3_753d5), d_V_f_SG_D_3_block/5(State_psi_d_SG_D_3_e6d3d), d_w_SG_D_3_block/3(State_psi_d_SG_D_3_195dc), i_q_SG_D_3_block/6(State_psi_d_SG_D_3_97c3b), T_e_SG_D_3_block/1(State_psi_d_SG_D_3_193a7), T_e_SG_D_3_block/7(State_psi_d_SG_D_3_dbbf4)
  v_d_SG_D_3/1 -> d_psi_d_SG_D_3_block/4(Input_v_d_SG_D_3_c1082), d_psi_q_SG_D_3_block/4(Input_v_d_SG_D_3_4ab93)
  v_q_SG_D_3/1 -> d_psi_d_SG_D_3_block/6(Input_v_q_SG_D_3_d2650), d_psi_q_SG_D_3_block/6(Input_v_q_SG_D_3_8644a)
  psi_q_SG_D_3/1 -> d_psi_d_SG_D_3_block/8(State_psi_q_SG_D_3_63db3), d_psi_q_SG_D_3_block/3(State_psi_q_SG_D_3_7832e), d_psi_gq_SG_D_3_block/6(State_psi_q_SG_D_3_af9de), d_psi_gq_SG_D_3_block/9(State_psi_q_SG_D_3_230f7), d_psi_kq_SG_D_3_block/5(State_psi_q_SG_D_3_2e3f0), d_w_SG_D_3_block/6(State_psi_q_SG_D_3_bf6de), d_w_SG_D_3_block/7(State_psi_q_SG_D_3_f5e8c), d_V_f_SG_D_3_block/7(State_psi_q_SG_D_3_af581), i_d_SG_D_3_block/3(State_psi_q_SG_D_3_a0a36), T_e_SG_D_3_block/4(State_psi_q_SG_D_3_a96b5), i_q_SG_D_3_block/3(State_psi_q_SG_D_3_7680a), T_e_SG_D_3_block/5(State_psi_q_SG_D_3_acbca), d_V_f_SG_D_3_block/11(State_psi_q_SG_D_3_590de)
  T_m_SG_D_3/1 -> d_T_m_SG_D_3_block/2(State_T_m_SG_D_3_a1980), d_w_SG_D_3_block/2(State_T_m_SG_D_3_662ce)
  T_e_SG_D_3_block/1(Blockout_T_e_SG_D_3_7d8b1) -> T_e_SG_D_3/1
  d_psi_d_SG_D_3_block/1(Blockout_d_psi_d_SG_D_3_12622) -> psi_d_SG_D_3/1
  i_d_SG_D_3_block/1(Blockout_i_d_SG_D_3_81b50) -> i_d_SG_D_3/1
  d_psi_gq_SG_D_3_block/1(Blockout_d_psi_gq_SG_D_3_a28a2) -> psi_gq_SG_D_3/1
  theta_SG_D_3_out_block/1(Blockout_theta_SG_D_3_out_f6982) -> theta_SG_D_3_out/1
  d_V_f_SG_D_3_block/1(Blockout_d_V_f_SG_D_3_fde33) -> V_f_SG_D_3/1
  d_R_f_SG_D_3_block/1(Blockout_d_R_f_SG_D_3_4784a) -> R_f_SG_D_3/1
  d_psi_q_SG_D_3_block/1(Blockout_d_psi_q_SG_D_3_417db) -> psi_q_SG_D_3/1
  i_q_SG_D_3_block/1(Blockout_i_q_SG_D_3_d02b0) -> i_q_SG_D_3/1
  d_psi_1d_SG_D_3_block/1(Blockout_d_psi_1d_SG_D_3_549d8) -> psi_1d_SG_D_3/1
  V_f_SG_D_3/1 -> d_V_f_SG_D_3_block/14(State_V_f_SG_D_3_d28c9), d_E_fd_SG_D_3_block/2(State_V_f_SG_D_3_2efed)
  Px_3_SG_D_3/1 -> d_V_f_SG_D_3_block/3(State_Px_3_SG_D_3_5d1f7), d_Px_3_SG_D_3_block/1(State_Px_3_SG_D_3_8aa31)
  d_E_fd_SG_D_3_block/1(Blockout_d_E_fd_SG_D_3_49225) -> E_fd_SG_D_3/1
  E_fd_SG_D_3/1 -> d_V_f_SG_D_3_block/1(State_E_fd_SG_D_3_f8a4b), d_E_fd_SG_D_3_block/1(State_E_fd_SG_D_3_4edb4), d_psi_fd_SG_D_3_block/1(State_E_fd_SG_D_3_68bde), d_R_f_SG_D_3_block/1(State_E_fd_SG_D_3_ddbea)
  d_psi_fd_SG_D_3_block/1(Blockout_d_psi_fd_SG_D_3_68982) -> psi_fd_SG_D_3/1

== system IEEE9_case/Subsystem ==
  uq : Inport
  ud : Inport  Port=2
  id : Inport  Port=3
  iq : Inport  Port=4
  Add : Sum
  Product : Product
  Product1 : Product
  Out1 : Outport
  wires:
  Product/1 -> Add/1
  id/1 -> Product/2
  ud/1 -> Product/1
  uq/1 -> Product1/1
  Product1/1 -> Add/2
  Add/1 -> Out1/1
  iq/1 -> Product1/2

== system IEEE9_case/Subsystem1 ==
  id : Inport
  iq : Inport  Port=2
  ud : Inport  Port=3
  uq : Inport  Port=4
  Add1 : Sum  Inputs=+-
  Product : Product
  Product1 : Product
  Out1 : Outport
  wires:
  Product1/1 -> Add1/2
  ud/1 -> Product1/2
  Add1/1 -> Out1/1
  Product/1 -> Add1/1
  iq/1 -> Product1/1
  id/1 -> Product/2
  uq/1 -> Product/1

== system IEEE9_case/Subsystem2 ==
  uq : Inport
  ud : Inport  Port=2
  id : Inport  Port=3
  iq : Inport  Port=4
  Add : Sum
  Product : Product
  Product1 : Product
  Out1 : Outport
  wires:
  Product/1 -> Add/1
  id/1 -> Product/2
  ud/1 -> Product/1
  uq/1 -> Product1/1
  Product1/1 -> Add/2
  Add/1 -> Out1/1
  iq/1 -> Product1/2

== system IEEE9_case/Subsystem3 ==
  id : Inport
  iq : Inport  Port=2
  ud : Inport  Port=3
  uq : Inport  Port=4
  Add1 : Sum  Inputs=+-
  Product : Product
  Product1 : Product
  Out1 : Outport
  wires:
  Product1/1 -> Add1/2
  ud/1 -> Product1/2
  Add1/1 -> Out1/1
  Product/1 -> Add1/1
  iq/1 -> Product1/1
  id/1 -> Product/2
  uq/1 -> Product/1

== system IEEE9_case/Subsystem4 ==
  id : Inport
  iq : Inport  Port=2
  uq : Inport  Port=3
  ud : Inport  Port=4
  Add1 : Sum  Inputs=+-
  Product : Product
  Product1 : Product
  Out1 : Outport
  wires:
  uq/1 -> Product/1
  id/1 -> Product/2
  iq/1 -> Product1/1
  Product/1 -> Add1/1
  Add1/1 -> Out1/1
  ud/1 -> Product1/2
  Product1/1 -> Add1/2

== system IEEE9_case/Subsystem5 ==
  uq : Inport
  ud : Inport  Port=2
  id : Inport  Port=3
  iq : Inport  Port=4
  Add : Sum
  Product : Product
  Product1 : Product
  Out1 : Outport
  wires:
  Product/1 -> Add/1
  id/1 -> Product/2
  ud/1 -> Product/1
  uq/1 -> Product1/1
  Product1/1 -> Add/2
  Add/1 -> Out1/1
  iq/1 -> Product1/2

== system IEEE9_case/Subsystem6 ==
  tt : Inport
  ft : Inport  Port=2
  tv : Inport  Port=3
  fv : Inport  Port=4
  Clock : Clock
  Minus : Sum  Inputs=+-
  Minus1 : Sum  Inputs=+-
  Switch : Switch  Criteria=u2 > Threshold  SaturateOnIntegerOverflow=off  InputSameDT=off
  Switch1 : Switch  Criteria=u2 > Threshold  SaturateOnIntegerOverflow=off  InputSameDT=off
  Out1 : Outport
  wires:
  ft/1 -> Minus/2
  Switch/1 -> Switch1/3
  Clock/1 -> Minus1/1, Minus/1
  Minus1/1 -> Switch1/2
  Switch1/1 -> Out1/1
  Minus/1 -> Switch/2
  fv/1 -> Switch1/1, Switch/3
  tt/1 -> Minus1/2
  tv/1 -> Switch/1

== system IEEE9_case/AC_1/d_id_line_1_4_block ==
  note: d_id_line_1_4 in IEEE9_case
      | $376.991118430775\,\mathrm{iq}_{\mathrm{line},1,4}+6544.98469497874\,\mathrm{vd}_{\mathrm{bus},1}-6544.98469497874\,\mathrm{vd}_{\mathrm{bus},4}$
      | Automatically generated on 2025-11-01 08:50:58 .
  State_iq_line_1_4_5b1cb : Inport
  State_vd_bus_1_9b5a0 : Inport  Port=2
  State_vd_bus_4_87ca3 : Inport  Port=3
  Add_562b3 : Sum
  Constant_376.991118430775_36767 : Constant  Value=376.991118430775
  Constant_6544.98469497874_70be5 : Constant  Value=6544.98469497874
  Constant_6544.98469497874_c704c : Constant  Value=6544.98469497874
  Product_48af5 : Product
  Product_93c34 : Product
  Product_a62e0 : Product
  Subtract_68bf6 : Sum  Inputs=+-
  Blockout_d_id_line_1_4_47f01 : Outport
  wires:
  Constant_376.991118430775_36767/1 -> Product_93c34/1
  Product_a62e0/1 -> Add_562b3/2
  State_iq_line_1_4_5b1cb/1 -> Product_93c34/2
  Subtract_68bf6/1 -> Blockout_d_id_line_1_4_47f01/1
  Constant_6544.98469497874_c704c/1 -> Product_a62e0/1
  Product_93c34/1 -> Add_562b3/1
  State_vd_bus_1_9b5a0/1 -> Product_a62e0/2
  Constant_6544.98469497874_70be5/1 -> Product_48af5/1
  State_vd_bus_4_87ca3/1 -> Product_48af5/2
  Add_562b3/1 -> Subtract_68bf6/1
  Product_48af5/1 -> Subtract_68bf6/2

== system IEEE9_case/AC_1/d_id_line_3_6_block ==
  note: d_id_line_3_6 in IEEE9_case
      | $376.991118430775\,\mathrm{iq}_{\mathrm{line},3,6}+6433.29553636135\,\mathrm{vd}_{\mathrm{bus},3}-6433.29553636135\,\mathrm{vd}_{\mathrm{bus},6}$
      | Automatically generated on 2025-11-01 08:51:04 .
  State_iq_line_3_6_057f5 : Inport
  State_vd_bus_3_1ec5f : Inport  Port=2
  State_vd_bus_6_a863a : Inport  Port=3
  Add_092c3 : Sum
  Constant_376.991118430775_4e5e5 : Constant  Value=376.991118430775
  Constant_6433.29553636135_6cdac : Constant  Value=6433.29553636135
  Constant_6433.29553636135_b1a29 : Constant  Value=6433.29553636135
  Product_2e6a1 : Product
  Product_c9e5d : Product
  Product_e8b5f : Product
  Subtract_46416 : Sum  Inputs=+-
  Blockout_d_id_line_3_6_e83e3 : Outport
  wires:
  State_vd_bus_3_1ec5f/1 -> Product_2e6a1/2
  Constant_376.991118430775_4e5e5/1 -> Product_e8b5f/1
  Product_2e6a1/1 -> Add_092c3/2
  State_iq_line_3_6_057f5/1 -> Product_e8b5f/2
  Constant_6433.29553636135_b1a29/1 -> Product_2e6a1/1
  Product_e8b5f/1 -> Add_092c3/1
  Constant_6433.29553636135_6cdac/1 -> Product_c9e5d/1
  State_vd_bus_6_a863a/1 -> Product_c9e5d/2
  Add_092c3/1 -> Subtract_46416/1
  Product_c9e5d/1 -> Subtract_46416/2
  Subtract_46416/1 -> Blockout_d_id_line_3_6_e83e3/1

== system IEEE9_case/AC_1/d_id_line_4_5_block ==
  note: d_id_line_4_5 in IEEE9_case
      | $376.991118430775\,\mathrm{iq}_{\mathrm{line},4,5}-69.6614023187302\,\mathrm{id}_{\mathrm{line},4,5}+4097.7295481606\,\mathrm{vd}_{\mathrm{bus},4}-4097.7295481606\,\mathrm{vd}_{\mathrm{bus},5}$
      | Automatically generated on 2025-11-01 08:51:00 .
  State_id_line_4_5_42986 : Inport
  State_iq_line_4_5_f0025 : Inport  Port=2
  State_vd_bus_4_0a732 : Inport  Port=3
  State_vd_bus_5_ce0e6 : Inport  Port=4
  Add_b9437 : Sum
  Add_f2bac : Sum
  Constant_-69.6614023187302_81780 : Constant  Value=-69.6614023187302
  Constant_376.991118430775_64b05 : Constant  Value=376.991118430775
  Constant_4097.7295481606_6bfbc : Constant  Value=4097.7295481606
  Constant_4097.7295481606_ae851 : Constant  Value=4097.7295481606
  Product_102bf : Product
  Product_64526 : Product
  Product_a0400 : Product
  Product_a87b4 : Product
  Subtract_4e9fa : Sum  Inputs=+-
  Blockout_d_id_line_4_5_192af : Outport
  wires:
  Constant_-69.6614023187302_81780/1 -> Product_64526/1
  Product_a87b4/1 -> Add_b9437/2
  State_id_line_4_5_42986/1 -> Product_64526/2
  Constant_376.991118430775_64b05/1 -> Product_a87b4/1
  State_iq_line_4_5_f0025/1 -> Product_a87b4/2
  Product_64526/1 -> Add_b9437/1
  Constant_4097.7295481606_ae851/1 -> Product_a0400/1
  State_vd_bus_4_0a732/1 -> Product_a0400/2
  Add_b9437/1 -> Add_f2bac/1
  Product_a0400/1 -> Add_f2bac/2
  Constant_4097.7295481606_6bfbc/1 -> Product_102bf/1
  State_vd_bus_5_ce0e6/1 -> Product_102bf/2
  Add_f2bac/1 -> Subtract_4e9fa/1
  Product_102bf/1 -> Subtract_4e9fa/2
  Subtract_4e9fa/1 -> Blockout_d_id_line_4_5_192af/1

== system IEEE9_case/AC_1/d_id_line_5_6_block ==
  note: d_id_line_5_6 in IEEE9_case
      | $376.991118430775\,\mathrm{iq}_{\mathrm{line},5,6}-86.4861977576484\,\mathrm{id}_{\mathrm{line},5,6}+2217.59481429868\,\mathrm{vd}_{\mathrm{bus},5}-2217.59481429868\,\mathrm{vd}_{\mathrm{bus},6}$
      | Automatically generated on 2025-11-01 08:51:02 .
  State_id_line_5_6_1a156 : Inport
  State_iq_line_5_6_e0044 : Inport  Port=2
  State_vd_bus_5_f7dd8 : Inport  Port=3
  State_vd_bus_6_81e43 : Inport  Port=4
  Add_4873d : Sum
  Add_de6f6 : Sum
  Constant_-86.4861977576484_f004d : Constant  Value=-86.4861977576484
  Constant_2217.59481429868_e06c4 : Constant  Value=2217.59481429868
  Constant_2217.59481429868_fd96a : Constant  Value=2217.59481429868
  Constant_376.991118430775_cf874 : Constant  Value=376.991118430775
  Product_22969 : Product
  Product_4b002 : Product
  Product_7fde0 : Product
  Product_f0704 : Product
  Subtract_24d58 : Sum  Inputs=+-
  Blockout_d_id_line_5_6_9f7f0 : Outport
  wires:
  Constant_-86.4861977576484_f004d/1 -> Product_f0704/1
  Product_7fde0/1 -> Add_4873d/2
  State_id_line_5_6_1a156/1 -> Product_f0704/2
  Constant_376.991118430775_cf874/1 -> Product_7fde0/1
  Product_f0704/1 -> Add_4873d/1
  State_iq_line_5_6_e0044/1 -> Product_7fde0/2
  Constant_2217.59481429868_fd96a/1 -> Product_4b002/1
  Product_22969/1 -> Subtract_24d58/2
  State_vd_bus_5_f7dd8/1 -> Product_4b002/2
  Add_4873d/1 -> Add_de6f6/1
  Product_4b002/1 -> Add_de6f6/2
  Constant_2217.59481429868_e06c4/1 -> Product_22969/1
  State_vd_bus_6_81e43/1 -> Product_22969/2
  Add_de6f6/1 -> Subtract_24d58/1
  Subtract_24d58/1 -> Blockout_d_id_line_5_6_9f7f0/1

== system IEEE9_case/AC_1/d_id_line_6_7_block ==
  note: d_id_line_6_7 in IEEE9_case
      | $376.991118430775\,\mathrm{iq}_{\mathrm{line},6,7}-44.5058959258554\,\mathrm{id}_{\mathrm{line},6,7}+3739.99125427356\,\mathrm{vd}_{\mathrm{bus},6}-3739.99125427356\,\mathrm{vd}_{\mathrm{bus},7}$
      | Automatically generated on 2025-11-01 08:51:07 .
  State_id_line_6_7_bd89c : Inport
  State_iq_line_6_7_bf0cc : Inport  Port=2
  State_vd_bus_6_1b476 : Inport  Port=3
  State_vd_bus_7_39ba6 : Inport  Port=4
  Add_6750f : Sum
  Add_7b6d1 : Sum
  Constant_-44.5058959258554_7828b : Constant  Value=-44.5058959258554
  Constant_3739.99125427356_3602a : Constant  Value=3739.99125427356
  Constant_3739.99125427356_51cc5 : Constant  Value=3739.99125427356
  Constant_376.991118430775_45a66 : Constant  Value=376.991118430775
  Product_21b31 : Product
  Product_487e7 : Product
  Product_aa508 : Product
  Product_c2205 : Product
  Subtract_8ca75 : Sum  Inputs=+-
  Blockout_d_id_line_6_7_12f87 : Outport
  wires:
  Constant_-44.5058959258554_7828b/1 -> Product_c2205/1
  Product_aa508/1 -> Add_6750f/2
  State_id_line_6_7_bd89c/1 -> Product_c2205/2
  Constant_376.991118430775_45a66/1 -> Product_aa508/1
  State_iq_line_6_7_bf0cc/1 -> Product_aa508/2
  Product_c2205/1 -> Add_6750f/1
  Constant_3739.99125427356_51cc5/1 -> Product_21b31/1
  State_vd_bus_6_1b476/1 -> Product_21b31/2
  Add_6750f/1 -> Add_7b6d1/1
  Product_21b31/1 -> Add_7b6d1/2
  Constant_3739.99125427356_3602a/1 -> Product_487e7/1
  State_vd_bus_7_39ba6/1 -> Product_487e7/2
  Add_7b6d1/1 -> Subtract_8ca75/1
  Product_487e7/1 -> Subtract_8ca75/2
  Subtract_8ca75/1 -> Blockout_d_id_line_6_7_12f87/1

== system IEEE9_case/AC_1/d_id_line_7_8_block ==
  note: d_id_line_7_8 in IEEE9_case
      | $376.991118430775\,\mathrm{iq}_{\mathrm{line},7,8}-44.5058959258554\,\mathrm{id}_{\mathrm{line},7,8}+5235.98775598299\,\mathrm{vd}_{\mathrm{bus},7}-5235.98775598299\,\mathrm{vd}_{\mathrm{bus},8}$
      | Automatically generated on 2025-11-01 08:51:09 .
  State_id_line_7_8_54820 : Inport
  State_iq_line_7_8_790f7 : Inport  Port=2
  State_vd_bus_7_19431 : Inport  Port=3
  State_vd_bus_8_e84a0 : Inport  Port=4
  Add_c6525 : Sum
  Add_d0411 : Sum
  Constant_-44.5058959258554_1691c : Constant  Value=-44.5058959258554
  Constant_376.991118430775_06e26 : Constant  Value=376.991118430775
  Constant_5235.98775598299_0136d : Constant  Value=5235.98775598299
  Constant_5235.98775598299_575e1 : Constant  Value=5235.98775598299
  Product_052f9 : Product
  Product_6daec : Product
  Product_b1821 : Product
  Product_dddb0 : Product
  Subtract_5a112 : Sum  Inputs=+-
  Blockout_d_id_line_7_8_47088 : Outport
  wires:
  Constant_-44.5058959258554_1691c/1 -> Product_6daec/1
  Product_b1821/1 -> Add_d0411/2
  State_id_line_7_8_54820/1 -> Product_6daec/2
  Constant_376.991118430775_06e26/1 -> Product_b1821/1
  Product_6daec/1 -> Add_d0411/1
  State_iq_line_7_8_790f7/1 -> Product_b1821/2
  Constant_5235.98775598299_0136d/1 -> Product_052f9/1
  State_vd_bus_7_19431/1 -> Product_052f9/2
  Add_d0411/1 -> Add_c6525/1
  Product_052f9/1 -> Add_c6525/2
  Constant_5235.98775598299_575e1/1 -> Product_dddb0/1
  State_vd_bus_8_e84a0/1 -> Product_dddb0/2
  Add_c6525/1 -> Subtract_5a112/1
  Product_dddb0/1 -> Subtract_5a112/2
  Subtract_5a112/1 -> Blockout_d_id_line_7_8_47088/1

== system IEEE9_case/AC_1/d_id_line_8_2_block ==
  note: d_id_line_8_2 in IEEE9_case
      | $376.991118430775\,\mathrm{iq}_{\mathrm{line},8,2}-6031.8578948924\,\mathrm{vd}_{\mathrm{bus},2}+6031.8578948924\,\mathrm{vd}_{\mathrm{bus},8}$
      | Automatically generated on 2025-11-01 08:51:11 .
  State_iq_line_8_2_9277c : Inport
  State_vd_bus_2_232dc : Inport  Port=2
  State_vd_bus_8_a337d : Inport  Port=3
  Add_9598a : Sum
  Constant_376.991118430775_49fff : Constant  Value=376.991118430775
  Constant_6031.8578948924_65ddc : Constant  Value=6031.8578948924
  Constant_6031.8578948924_b24d8 : Constant  Value=6031.8578948924
  Product_1ebbd : Product
  Product_afef8 : Product
  Product_fafd4 : Product
  Subtract_c7711 : Sum  Inputs=+-
  Blockout_d_id_line_8_2_95461 : Outport
  wires:
  State_vd_bus_2_232dc/1 -> Product_afef8/2
  Constant_376.991118430775_49fff/1 -> Product_1ebbd/1
  Product_afef8/1 -> Subtract_c7711/2
  State_iq_line_8_2_9277c/1 -> Product_1ebbd/2
  Constant_6031.8578948924_b24d8/1 -> Product_afef8/1
  Product_1ebbd/1 -> Subtract_c7711/1
  Constant_6031.8578948924_65ddc/1 -> Product_fafd4/1
  State_vd_bus_8_a337d/1 -> Product_fafd4/2
  Subtract_c7711/1 -> Add_9598a/1
  Product_fafd4/1 -> Add_9598a/2
  Add_9598a/1 -> Blockout_d_id_line_8_2_95461/1

== system IEEE9_case/AC_1/d_id_line_8_9_block ==
  note: d_id_line_8_9 in IEEE9_case
      | $376.991118430775\,\mathrm{iq}_{\mathrm{line},8,9}-74.9299117377938\,\mathrm{id}_{\mathrm{line},8,9}+2341.55974180606\,\mathrm{vd}_{\mathrm{bus},8}-2341.55974180606\,\mathrm{vd}_{\mathrm{bus},9}$
      | Automatically generated on 2025-11-01 08:51:13 .
  State_id_line_8_9_588f7 : Inport
  State_iq_line_8_9_a71ff : Inport  Port=2
  State_vd_bus_8_8f873 : Inport  Port=3
  State_vd_bus_9_4af5d : Inport  Port=4
  Add_6c052 : Sum
  Add_f75f3 : Sum
  Constant_-74.9299117377938_ec2dd : Constant  Value=-74.9299117377938
  Constant_2341.55974180606_458bb : Constant  Value=2341.55974180606
  Constant_2341.55974180606_49cb8 : Constant  Value=2341.55974180606
  Constant_376.991118430775_d8afd : Constant  Value=376.991118430775
  Product_a0be3 : Product
  Product_e765e : Product
  Product_e8b47 : Product
  Product_f085f : Product
  Subtract_ca8cf : Sum  Inputs=+-
  Blockout_d_id_line_8_9_1db1d : Outport
  wires:
  Constant_-74.9299117377938_ec2dd/1 -> Product_e8b47/1
  Product_a0be3/1 -> Add_f75f3/2
  State_id_line_8_9_588f7/1 -> Product_e8b47/2
  Constant_376.991118430775_d8afd/1 -> Product_a0be3/1
  State_iq_line_8_9_a71ff/1 -> Product_a0be3/2
  Product_e8b47/1 -> Add_f75f3/1
  Constant_2341.55974180606_458bb/1 -> Product_f085f/1
  State_vd_bus_8_8f873/1 -> Product_f085f/2
  Add_f75f3/1 -> Add_6c052/1
  Product_f085f/1 -> Add_6c052/2
  Constant_2341.55974180606_49cb8/1 -> Product_e765e/1
  State_vd_bus_9_4af5d/1 -> Product_e765e/2
  Add_6c052/1 -> Subtract_ca8cf/1
  Product_e765e/1 -> Subtract_ca8cf/2
  Subtract_ca8cf/1 -> Blockout_d_id_line_8_9_1db1d/1
